simulink model "sim_gs_sat"  (R2024a)
settings: Solver=FixedStepAuto  StartTime=0.0  StopTime=150.0  FixedStep=1e-3  RelTol=1e-3
InitFcn:
  | T=0.01;
settings Model: Creator=alexe  LastModifiedBy=alexe

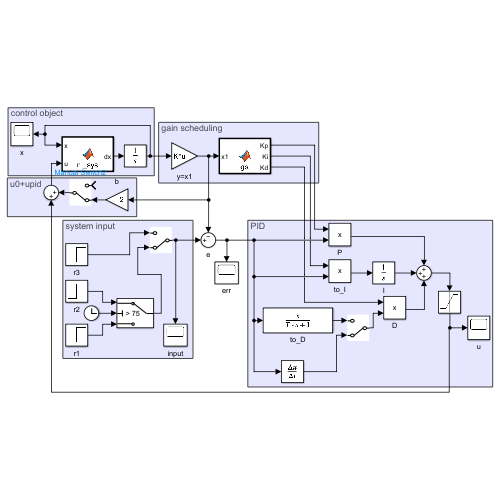
[thumbnail: Simulink's stored preview of the top-level diagram]
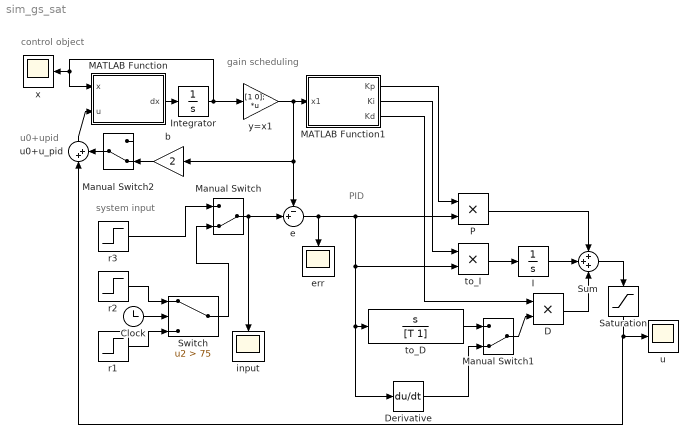
== system sim_gs_sat ==
  note: u0+upid
  note: system input
  note: control object
  note: gain scheduling
  note: PID
  Clock : Clock
  D : Product
  Derivative : Derivative
  I : Integrator
  Integrator : Integrator  InitialCondition=[0;0];
  MATLAB Function : MATLAB Function  TreatAsAtomicUnit=on
  MATLAB Function1 : MATLAB Function  TreatAsAtomicUnit=on
  Manual Switch : ManualSwitch  CurrentSetting=0
  Manual Switch1 : ManualSwitch  CurrentSetting=0
  Manual Switch2 : ManualSwitch  CurrentSetting=0
  P : Product
  Saturation : Saturate  UpperLimit=10  LowerLimit=-10
  Sum : Sum  Inputs=+++
  Switch : Switch  Criteria=u2 > Threshold  Threshold=75  SaturateOnIntegerOverflow=off  InputSameDT=off
  b : Gain  Gain=2
  e : Sum  Inputs=-+|
  err : Scope
  input : Scope
  r1 : Step  Time=25  Before=1  After=2  SampleTime=0
  r2 : Step  Time=0  Before=2  After=3  SampleTime=0
  r3 : Step  Time=25  Before=1  After=3  SampleTime=0
  to_D : TransferFcn  Numerator=[1 0]  Denominator=[T 1]
  to_I : Product
  u : Scope
  u0+u_pid : Sum  Inputs=|++
  x : Scope
  y=x1 : Gain  Gain=[1 0];  Multiplication=Matrix(K*u)
  wires:
  y=x1/1 -> MATLAB Function1/1(x1), e/1, b/1
  MATLAB Function1/1(Kp) -> P/1
  e/1 -> err/1, P/2, to_I/2, to_D/1, Derivative/1
  MATLAB Function1/2(Ki) -> to_I/1
  to_I/1 -> I/1
  MATLAB Function1/3(Kd) -> D/1
  I/1 -> Sum/2
  P/1 -> Sum/1
  Integrator/1 -> y=x1/1, MATLAB Function/1(x), x/1
  Clock/1 -> Switch/2
  r2/1 -> Switch/1
  r1/1 -> Switch/3
  Sum/1 -> Saturation/1
  D/1 -> Sum/3
  u0+u_pid/1 -> MATLAB Function/2(u)
  Manual Switch/1 -> input/1, e/2
  r3/1 -> Manual Switch/1
  Switch/1 -> Manual Switch/2
  Manual Switch1/1 -> D/2
  to_D/1 -> Manual Switch1/1
  Derivative/1 -> Manual Switch1/2
  MATLAB Function/1(dx) -> Integrator/1
  Saturation/1 -> u0+u_pid/1, u/1
  Manual Switch2/1 -> u0+u_pid/2
  b/1 -> Manual Switch2/2

== matlab function sim_gs_sat/MATLAB Function ==
  data: x input; u input; dx output
function dx = nl_sys(x,u)

a0 = 0.5;
a1 = 1.3;
b  = 2;

a = a0 + a1*x(1)^2;

dx = zeros(2,1);
dx(1) = x(2);
dx(2) = -a*x(2) - b*x(1) + u;

== matlab function sim_gs_sat/MATLAB Function1 ==
  data: x1 input; Kp output; Ki output; Kd output
function [Kp,Ki,Kd] = gs(x1)

if abs(x1) < 1.5
    Kp=4.39;
    Ki=4.07;
    Kd=1.19;
elseif abs(x1) < 2.5
    Kp=3.16;
    Ki=1.97;
    Kd=0.72;
else
    Kp=2.75;
    Ki=0.92;
    Kd=0.00;
end
